simulink model "nnetInferenceTest"  (R2020b)
settings: Solver=FixedStepDiscrete  StartTime=0.0  StopTime=stopTime  RelTol=1e-3
PostLoadFcn:
  | addpath([fileparts(which(bdroot)) filesep '..' filesep])
  | simulinkNnetPostLoadCallback
InitFcn:
  | simulinkInitNnetInference
StopFcn:
  | simulinkVerifyNnetInference
undefined symbols (not defined in the file or in its folder): params
libraries: dspsrcs4 x1
settings Model: DataTypeOverride=Off  SimulationMode=accelerator  PauseTimes=1  Creator=trevor  LastModifiedBy=trevor
settings DataIOCC: SaveOutput=off  DSMLogging=off  SaveTime=off  ReturnWorkspaceOutputs=off
settings OptimizationCC: BlockReduction=off  ConditionallyExecuteInputs=off  DefaultParameterBehavior=Inlined
settings DebuggingCC: AlgebraicLoopMsg=error  SingleTaskRateTransMsg=error  SFMachineParentedDataDiag=error
settings HardwareCC: ProdBitPerPointer=32  ProdBitPerSizeT=32  ProdBitPerPtrDiffT=32  ProdLargestAtomicFloat=None  ProdIntDivRoundTo=Undefined  ProdEndianess=Unspecified  ProdWordSize=32  ProdHWDeviceType=ASIC/FPGA->ASIC/FPGA  TargetBitPerLong=64  TargetBitPerPointer=64  TargetBitPerSizeT=64  TargetBitPerPtrDiffT=64  TargetLongLongMode=on  TargetIntDivRoundTo=Zero  TargetEndianess=LittleEndian  TargetWordSize=64  TargetHWDeviceType=Custom Processor->MATLAB Host Computer  ProdEqTarget=off

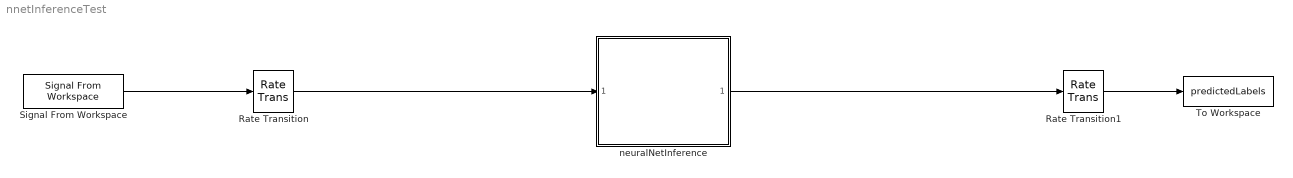
== system nnetInferenceTest ==
  Rate Transition : RateTransition  Deterministic=off  OutPortSampleTime=params.systemClockPeriod
  Rate Transition1 : RateTransition  Deterministic=off  OutPortSampleTime=params.samplingPeriod
  Signal From Workspace : dspsrcs4/Signal From Workspace  X=inputFeatures  Ts=params.samplingPeriod  nsamps=1  OutputAfterFinalValue=Setting to zero  ignoreOrWarnInputAndFrameLengths=off  OutputFrames=off
  To Workspace : ToWorkspace  VariableName=predictedLabels  SampleTime=-1
      settings: Save2DSignal=2-D array (concatenate along first dimension)
  neuralNetInference : Subsystem  ReferencedSubsystem=neuralNetInference
  wires:
  Signal From Workspace/1 -> Rate Transition/1
  Rate Transition1/1 -> To Workspace/1
  Rate Transition/1 -> neuralNetInference/1
  neuralNetInference/1 -> Rate Transition1/1
